simulink model "Inverse7Joint"  (R2023a)
settings: Solver=VariableStepAuto  StartTime=0.0  StopTime=240  RelTol=1e-3
libraries: dspnetwork x2, sldrtlib x1
settings Model: Creator=dr  LastModifiedBy=jeric
settings DebuggingCC: UnconnectedInputMsg=warning  UnconnectedOutputMsg=warning  UnconnectedLineMsg=warning
settings ModelReferenceCC: EnableRefExpFcnMdlSchedulingChecks=on
settings RTWCC: DLArmComputeVersion=19.05

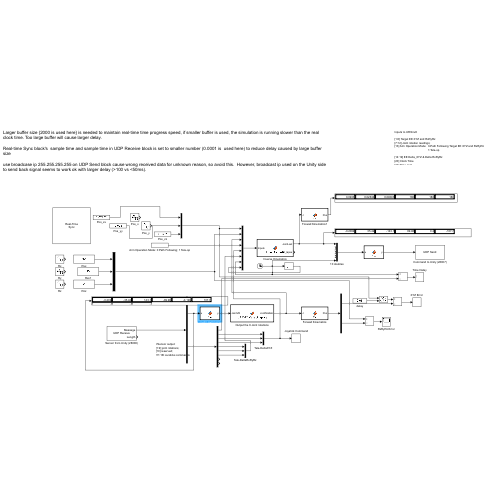
[thumbnail: Simulink's stored preview of the top-level diagram]
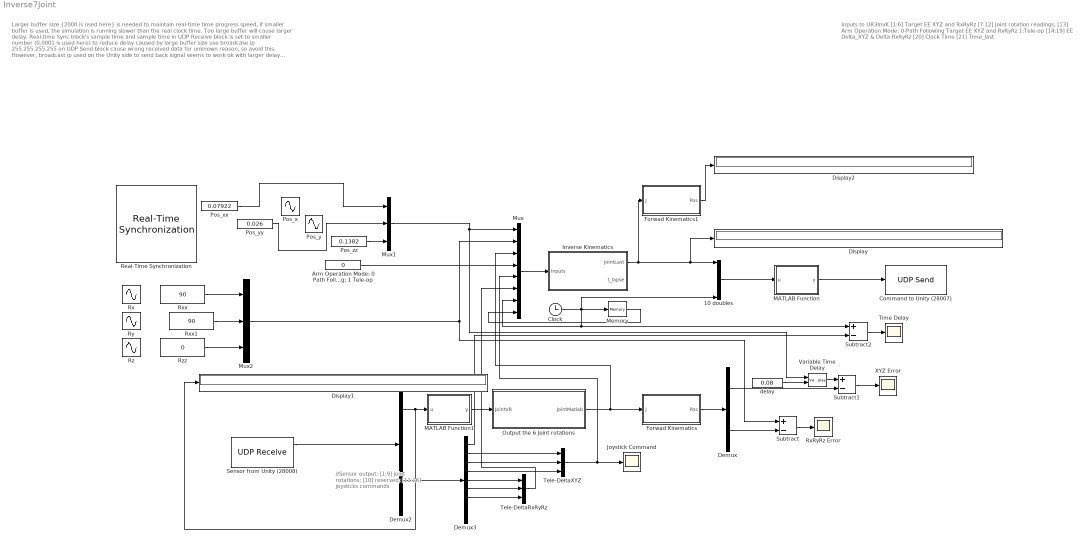
== system Inverse7Joint ==
  note: //Sensor output:
      | [1:9] joint rotations;
      | [10] reserved;
      | [11:16] joysticks commands
  note: Larger buffer size {2000 is used here} is needed to maintain real-time time progress speed, if smaller buffer is used, the simulation is running slower than the real clock time. Too large buffer will cause larger delay.
      |
      | Real-time Sync block's sample time and sample time in UDP Receive block is set to smaller number (0.0001 is used here) to reduce delay caused by large buffer size
      |
      | use broadcase ip 255.255.255.255 on UDP Send block cause wrong received data for unknown reason, so avoid this. However, broadcast ip used on the Unity side to send back signal seems to work ok with larger delay (>100 vs <50ms).
  note: Inputs to UR3InvK
      |
      | [1:6] Target EE XYZ and RxRyRz
      | [7:12] Joint rotation readings;
      | [13] Arm Operation Mode: 	0-Path Following Target EE XYZ and RxRyRz
      | 						1:Tele-op
      |
      | [14:19] EE Delta_XYZ & Delta RxRyRz
      | [20] Clock Time
      | [21] Time_last
  " Joystick Command" : Scope
  10 doubles : Mux  Inputs=5
  Arm Operation Mode: 0 Path Following; 1 Tele-op : Constant  Value=0
  Clock : Clock
  Command to Unity (28007) : dspnetwork/UDP Send  remoteURL='127.0.0.1'  remotePort=28007  localURL='0.0.0.0'  localPortSource=Automatically determine  localPort=-1  sendBufferSize=2500  sampletime=-1  blockPlatform=[]  separateLengthPort=0
  Demux : Demux  Outputs=2
  Demux2 : Demux  Outputs=2
  Demux3 : Demux  Outputs=9
  Display : Display
  Display1 : Display
  Display2 : Display
  Forwad Kinematics : MATLAB Function  TreatAsAtomicUnit=on
  Forwad Kinematics1 : MATLAB Function  TreatAsAtomicUnit=on
  Inverse Kinematics : MATLAB Function  TreatAsAtomicUnit=on
  MATLAB Function : MATLAB Function  TreatAsAtomicUnit=on
  MATLAB Function1 : MATLAB Function  TreatAsAtomicUnit=on
  Memory : Memory  InheritSampleTime=on
  Mux : Mux  Inputs=8
  Mux1 : Mux  Inputs=3
  Mux2 : Mux  Inputs=3
  Output the 6 Joint rotations : MATLAB Function  TreatAsAtomicUnit=on
  Pos_x : Sin  Amplitude=0.15  Bias=.38  Frequency=.0785  Phase=1.57  SampleTime=0.001
  Pos_xx : Constant  Value=0.07922
  Pos_y : Sin  Amplitude=0.2  Frequency=.0785  SampleTime=0.001
  Pos_yy : Constant  Value=0.026
  Pos_zz : Constant  Value=0.1382
  Real-Time Synchronization : sldrtlib/Real-Time Synchronization  SampleTime=0.0001  MaxMissedTicks=10000000  ShowMissedTicks=off  YieldWhenWaiting=on
  Rx : Sin  Amplitude=45  Bias=180  Frequency=.5  SampleTime=0.001
  RxRyRz Error : Scope
  Rxx : Constant  Value=90
  Rxx1 : Constant  Value=90
  Ry : Sin  Amplitude=45  Frequency=.5  SampleTime=0.001
  Rz : Sin  Amplitude=180  Bias=-90  Frequency=1.57  SampleTime=0.001
  Rzz : Constant  Value=0
  Sensor from Unity (28008) : dspnetwork/UDP Receive  localURL='0.0.0.0'  localPort=28008  remoteURL='127.0.0.1'  remotePort=-1  recvBufferSize=2500  dims=18  signalDatatype=double  isComplex=off  isVarSize=off  showBlockingTime=off  blockingTime=0  sampletime=0.0001  blockPlatform=[]
  Subtract : Sum  Inputs=+-
  Subtract1 : Sum  Inputs=+-
  Subtract2 : Sum  Inputs=+-
  Tele-DeltaRxRyRz : Mux  Inputs=3
  Tele-DeltaXYZ : Mux  Inputs=3
  Time Delay : Scope
  Variable Time Delay : VariableTransportDelay  MaximumDelay=10
  XYZ Error : Scope
  delay : Constant  Value=0.08
  wires:
  Mux/1 -> Inverse Kinematics/1(Inputs)
  Subtract/1 -> RxRyRz Error/1
  Output the 6 Joint rotations/1(JointMatlab) -> Mux/3, Forwad Kinematics/1(J)
  Demux/2 -> Subtract/2
  Demux/1 -> Subtract1/2
  Subtract1/1 -> XYZ Error/1
  Mux2/1 -> Mux/2, Subtract/1
  Forwad Kinematics/1(Pos) -> Demux/1
  Clock/1 -> 10 doubles/5, Mux/7, Subtract2/1, Memory/1
  Memory/1 -> Mux/8
  Rxx/1 -> Mux2/1
  Rzz/1 -> Mux2/3
  Mux1/1 -> Variable Time Delay/1, Mux/1
  Sensor from Unity (28008)/1 -> Demux2/1
  Demux2/2 -> Demux3/1
  Demux3/2 -> Tele-DeltaXYZ/1
  Demux3/3 -> Tele-DeltaXYZ/2
  Demux3/4 -> Tele-DeltaXYZ/3
  Demux3/5 -> Tele-DeltaRxRyRz/1
  Demux3/6 -> Tele-DeltaRxRyRz/2
  Demux3/7 -> Tele-DeltaRxRyRz/3
  Tele-DeltaXYZ/1 -> " Joystick Command"/1, Mux/5
  Arm Operation Mode: 0 Path Following; 1 Tele-op/1 -> Mux/4
  Tele-DeltaRxRyRz/1 -> Mux/6
  Subtract2/1 -> Time Delay/1
  Demux3/1 -> Subtract2/2
  Variable Time Delay/1 -> Subtract1/1
  delay/1 -> Variable Time Delay/2
  Rxx1/1 -> Mux2/2
  Pos_zz/1 -> Mux1/3
  Pos_xx/1 -> Mux1/1
  Pos_yy/1 -> Mux1/2
  Forwad Kinematics1/1(Pos) -> Display2/1
  Inverse Kinematics/1(JointLast) -> Forwad Kinematics1/1(J), Display/1, 10 doubles/1
  Demux2/1 -> MATLAB Function1/1(u), Display1/1
  10 doubles/1 -> MATLAB Function/1(u)
  MATLAB Function/1(y) -> Command to Unity (28007)/1
  MATLAB Function1/1(y) -> Output the 6 Joint rotations/1(JointVR)

== matlab function Inverse7Joint/Forwad Kinematics ==
  data: J input; Pos output

function Pos = FK(J)
    Joint = zeros(7,1);
    Pos = zeros(6,1);

    D2R = pi/180;

    for i = 1:6
        Joint(i) = J(i)*D2R;
    end
    Joint(7) = J(7);
    PTool = [0;0;-0.068;1];
    
    dh = [pi 0 0 Joint(1);
          pi/2 0 0 Joint(2);
          0 0.19538 0 Joint(3);
          0 0.16737 -0.0025 Joint(4);
          -pi/2 0 -0.05 Joint(5);
          -pi/2 0 -0.0285 Joint(6)];

 
    T=[1 0 0 0;0 1 0 0; 0 0 1 0; 0 0 0 1];

    for i = 1:6
        T = T*[cos(dh(i,4))              -sin(dh(i,4))             0             dh(i,2);
               sin(dh(i,4))*cos(dh(i,1)) cos(dh(i,4))*cos(dh(i,1)) -sin(dh(i,1)) -sin(dh(i,1))*dh(i,3);
               sin(dh(i,4))*sin(dh(i,1)) cos(dh(i,4))*sin(dh(i,1)) cos(dh(i,1))  cos(dh(i,1))*dh(i,3);
               0                         0                         0             1];
    end
    PTemp = T*PTool;
    Pos(1:3) = PTemp(1:3);

    Pos(4:6) = R2FA(T(1:3,1:3));
    Pos(4:6) = Pos(4:6)/D2R;

function [AX, AY, AZ] = R2FA(R)
    M = 0.0001;
    AY= atan2(-R(3,1), sqrt(R(1,1)^2+R(2,1)^2));
    CAY = cos(AY);

    if abs(CAY)>M
        AZ=atan2(R(2,1)/CAY, R(1,1)/CAY);
        AX=atan2(R(3,2)/CAY, R(3,3)/CAY);
    elseif AY>0
       AY=pi/2;
       AZ=0;
       AX=atan2(R(1,2), R(2,2));
    else
       AY=-pi/2;
       AZ=0; 
       AX=-atan2(R(1,2), R(2,2));
end

== matlab function Inverse7Joint/Forwad Kinematics1 ==
  data: J input; Pos output

function Pos = FK(J)
    Joint = zeros(7,1);
    Pos = zeros(6,1);

    D2R = pi/180;

    for i = 1:6
        Joint(i) = J(i)*D2R;
    end
    Joint(7) = J(7);
    PTool = [0;0;-0.068;1];
    
    dh = [pi 0 0 Joint(1);
          pi/2 0 0 Joint(2);
          0 0.19538 0 Joint(3);
          0 0.16737 -0.0025 Joint(4);
          -pi/2 0 -0.05 Joint(5);
          -pi/2 0 -0.0285 Joint(6)];

 
    T=[1 0 0 0;0 1 0 0; 0 0 1 0; 0 0 0 1];

    for i = 1:6
        T = T*[cos(dh(i,4))              -sin(dh(i,4))             0             dh(i,2);
               sin(dh(i,4))*cos(dh(i,1)) cos(dh(i,4))*cos(dh(i,1)) -sin(dh(i,1)) -sin(dh(i,1))*dh(i,3);
               sin(dh(i,4))*sin(dh(i,1)) cos(dh(i,4))*sin(dh(i,1)) cos(dh(i,1))  cos(dh(i,1))*dh(i,3);
               0                         0                         0             1];
    end
    PTemp = T*PTool;
    Pos(1:3) = PTemp(1:3);

    Pos(4:6) = R2FA(T(1:3,1:3));
    Pos(4:6) = Pos(4:6)/D2R;

function [AX, AY, AZ] = R2FA(R)
    M = 0.0001;
    AY= atan2(-R(3,1), sqrt(R(1,1)^2+R(2,1)^2));
    CAY = cos(AY);

    if abs(CAY)>M
        AZ=atan2(R(2,1)/CAY, R(1,1)/CAY);
        AX=atan2(R(3,2)/CAY, R(3,3)/CAY);
    elseif AY>0
       AY=pi/2;
       AZ=0;
       AX=atan2(R(1,2), R(2,2));
    else
       AY=-pi/2;
       AZ=0; 
       AX=-atan2(R(1,2), R(2,2));
end

== matlab function Inverse7Joint/Inverse Kinematics ==
  data: Inputs input; JointLast output; t_lapse output
function [JointLast, t_lapse]  = LunarArmInvK (Inputs)
persistent  PositionLast  RotationLast;

if isempty(PositionLast)
    PositionLast =zeros(3,1);
end

if isempty(RotationLast)
    RotationLast =zeros(3,1);
end

 
t_lapse = Inputs(20)- Inputs(21);

if Inputs(20) > 0.0 % delay start to make sure sensor data from the VR robot has arrived, during delay, send out the initial joint position 
 
% LEFT  ARM
% This function will generate the joint angle set for each joint on left
% arm based on drawing a circle on XZ plane, radius is RD.
% there are many import parameters is based on physical arm dimensions.
% please contact Dr Robot Inc for further information.

% The demo code is just for 'demo' use.

%cal Jacobian using 5.1.27, page 115, Robot Dyn and Control by Spong
%JInit

steps=5; 

Joint = zeros(6,steps+1);
JointWS = zeros(6,2);
Origin = zeros(3,6);
Axis = zeros(3,6);
PEnd = zeros (3,steps);
Jaco = zeros (6,6);
PTarget = zeros(3, steps+1);
FATarget = zeros(3, steps+1);
ODelta = zeros(3,steps);
WJointLtd = zeros (6,6);
JointLast = zeros (6,1);
RTeleDelta = eye(3,3);
finalPos = zeros(3,1);
finalRxRyRz = zeros(3,1);
PTeleDelta = zeros (3,1);  
Degree2Radian = pi/180;
RxRyRzTeleDelta = zeros(3,1);
RJ5 = zeros(3,3);

%initial joint position
Joint(1,1)= Inputs(7)*Degree2Radian;
Joint(2,1)= Inputs(8)*Degree2Radian;
Joint(3,1)= Inputs(9)*Degree2Radian;
Joint(4,1)= Inputs(10)*Degree2Radian;
Joint(5,1)= Inputs(11)*Degree2Radian;
Joint(6,1)= Inputs(12)*Degree2Radian;

%########################physical dimensions #############################
%Joint limit in degrees
JointLtd=[  -180,   180;
             -205,   25;
            -160,   160;
            -180,   180;
            -180,   180;
            -180,   180];
JointLtdExRate = 50; %Joint ltd avoidance exp increase rate, if this rate is too small, e.g. 10 or 1, it may exceed the limit a bit; 
JointSB=20; % safe zone before reaching joint limit, joint limit avoidance scheme starts action when entering the safe zone. effect grows exponentially
%Convert the safe operation zone (with a boundary of JointSB before the
%limit) from degree into the RAD
for i=1:6
           JointWS(i,1)=(JointLtd(i,1)+JointSB)*Degree2Radian;
           JointWS(i,2)=(JointLtd(i,2)-JointSB)*Degree2Radian;
end
       
T=[1 0 0 0;0 1 0 0; 0 0 1 0; 0 0 0 1]; %INITIAL  Transformation matrix
PTool=[0;0;-0.068;1]; %The Tool or tip position expressed wrt the last frame physical dimension
%Catisian space task weighting, i.e. position and orientation tracking task
%weight, smaller , less significant to track, i.e. by setting WEnd(4,4)
%smaller (e.g. 0.01 while others are 1), the rotation along RX axis will not be tracked precisely.
%!!!!!!!!!!!!!!!!!!!!CHANGE HERE

WEnd=[1 0 0 0 0 0;
    0 1 0 0 0 0;
    0 0 1 0 0 0;
    0 0 0 1 0 0;
    0 0 0 0 1 0;
    0 0 0 0 0 1];           %0.01

%Joint space weighting matrix, larger number will reduce the joint motion,
%i.e. the unit WJoint(6,6)=100, while others are "1" then the joint 6 will
%move very little.
%!!!!!!!!!!!!!!!!!!!!CHANGE HERE
% WJoint=[0.1 0 0 0 0 0;
%         0 0.1 0 0 0 0;
%         0 0 0.1 0 0 0;
%         0 0 0 1 0 0;
%         0 0 0 0 1 0;
%         0 0 0 0 0 1];
WJoint=[1 0 0 0 0 0;
        0 1 0 0 0 0;
        0 0 1 0 0 0;
        0 0 0 1 0 0;
        0 0 0 0 1 0;
        0 0 0 0 0 1];

 
DF2= 0.001; %0.15; %.015; %Damping factor square, larger, slower tracking, bigger tracking error, but more robust to singularity 


for k = 1:steps

    dh = [   pi              0           0           Joint(1,k); 
             pi/2           0           0           Joint(2,k);
             0              0.19538       0           Joint(3,k);
             0              0.16737       -0.0025           Joint(4,k);
             -pi/2            0           -0.05     Joint(5,k);
             -pi/2           0           -0.0285     Joint(6,k)];
 
T=[1 0 0 0;0 1 0 0; 0 0 1 0; 0 0 0 1]; %INITIAL  Transformation matrix

for m=1:6
T=T*[cos(dh(m,4))                    -sin(dh(m,4))                0               dh(m,2)
    sin(dh(m,4))*cos(dh(m,1))   cos(dh(m,4))*cos(dh(m,1))   -sin(dh(m,1))       -sin(dh(m,1))*dh(m,3)
    sin(dh(m,4))*sin(dh(m,1))   cos(dh(m,4))*sin(dh(m,1))   cos(dh(m,1))       cos(dh(m,1))*dh(m,3)
    0                               0                           0               1];
Axis(1:3,m)=T(1:3,3);
Origin(1:3,m)= T(1:3,4);
%if m==5 % copy the second last joint, (before the hand) Rotation
%    RJ5 = T(1:3,1:3);
%end

end

PEndTemp=T*PTool;
PEnd(1:3,k)=PEndTemp(1:3); %tip position in origin frame

%Jacobian upper part , i.e. the linear velocity part
Jaco(1:3,1)= cross (Axis (1:3,1), (PEnd (1:3,k) - Origin(1:3,1)));
Jaco(1:3,2)= cross (Axis (1:3,2), (PEnd (1:3,k)- Origin(1:3,2)));
Jaco(1:3,3)= cross (Axis (1:3,3), (PEnd (1:3,k)- Origin(1:3,3)));
Jaco(1:3,4)= cross (Axis (1:3,4), (PEnd (1:3,k)- Origin(1:3,4)));
Jaco(1:3,5)= cross (Axis (1:3,5), (PEnd (1:3,k)- Origin(1:3,5)));
Jaco(1:3,6)= cross (Axis (1:3,6), (PEnd (1:3,k)- Origin(1:3,6)));

%Jacobian lower part , i.e. the angular velocity part
Jaco(4:6,1)= Axis (1:3,1);
Jaco(4:6,2)= Axis (1:3,2);
Jaco(4:6,3)= Axis (1:3,3);
Jaco(4:6,4)= Axis (1:3,4);
Jaco(4:6,5)= Axis (1:3,5);
Jaco(4:6,6)= Axis (1:3,6);

if k==1 %cal the initial posotition and orientation from the initial joint reading
%target position, should use the sensor reading to calculate the X,Y,Z and
%plan the end effector motion accordingly to avoid rapid movement at start

PInitial    = PEnd(1:3,1);
RInitial    = T(1:3,1:3);
    
%Initialize the tip motion Target 
PTarget(1, 1) = PInitial(1);
PTarget(2, 1) = PInitial(2);
PTarget(3, 1) = PInitial(3) ;

InitialRxRyRZ=R2FixAngle(RInitial);
 
FATarget(1:3,1) = InitialRxRyRZ; %using Fixed-Angle representation page 47, intro to robotics

% set the final target position and RxRyRz
    if Inputs(13) >=1 % 1: tele-operation on end-effector, using Mode switching Initial pos + delat pos as the final target 
        magPosCommand = norm(Inputs(14:16));
        magRotCommand = norm(Inputs(17:19)); 

     if magPosCommand < 0.2  %no motion needed
         PTeleDelta = zeros(3,1);
     else
         PTeleDelta =RInitial*Inputs(14:16)*t_lapse*0.1;
     end

     if magRotCommand < 0.2 %no rotation needed
        RTeleDelta = eye(3,3);
     else
        RxRyRzTeleDelta = Inputs(17:19)*t_lapse*0.5;
        RTeleDelta = FixAngle2R (RxRyRzTeleDelta(1:3));   
     end
        
        finalPos = PositionLast + PTeleDelta;
        finalRxRyRz=R2FixAngle(FixAngle2R(RotationLast*Degree2Radian)*RTeleDelta)*180/pi;
        %finalRxRyRz = Inputs (4:6);
     
    else % =0 path following
        finalPos = Inputs (1:3);
        finalRxRyRz = Inputs (4:6);
    end
end    


%linear planning 
PTarget(1, k+1) = PTarget(1,1) + (finalPos(1)-PTarget(1,1))/steps*k;
PTarget(2, k+1) = PTarget(2,1) + (finalPos(2)-PTarget(2,1))/steps*k ;
PTarget(3, k+1) = PTarget(3,1) + (finalPos(3)-PTarget(3,1))/steps*k;
%PTarget(3, k+1) = PTarget(3,1) - RD - RD*cos(pi+ 2*pi*k/steps);


%planning the orientation motion

FATarget(1,k+1)= finalRxRyRz(1)*Degree2Radian ; 
FATarget(2,k+1)= finalRxRyRz(2)*Degree2Radian ;
FATarget(3,k+1)= finalRxRyRz(3)*Degree2Radian ;

RTarget = FixAngle2R(FATarget(1:3,k+1));

%tip motion delta
PDelta= PTarget(1:3,k+1)-PEnd(1:3,k);
%Rotation error
Rerror = RTarget*(T(1:3,1:3)');
ODelta(1:3,k) = 0.5*[Rerror(3,2)-Rerror(2,3); Rerror(1,3)-Rerror(3,1);Rerror(2,1)-Rerror(1,2)];

%Least square pseudo inverse of J
JacoP=Jaco(1:6,1:6);
%Jw=transpose(JacoP)*inv(JacoP*transpose(JacoP)+ DF2*eye(6));


%Joint limit avoidance
for i=1:6
    if Joint(i,k)>JointWS(i,2)
        JointOver= Joint(i,k)-JointWS(i,2);
    elseif     Joint(i,k) <JointWS(i,1)
        JointOver= JointWS(i,1)-Joint(i,k) ;
    else
       JointOver=0;     
   end   
WJointLtd(i,i)=WJoint(i,i)*exp(JointLtdExRate*JointOver); %Augment the WJoint weighting matrix with the Joint Limit Avoidance, closer to the limit, the Weighting unit will increase exponentially, and leading to smaller velocity till stop, therefore avoiding exceeding the limit
end

Jw=inv(transpose(JacoP)*WEnd*JacoP+ DF2*(WJointLtd))*transpose(JacoP)*WEnd;

%conJ=cond(JacoP)
%Jw=inv(Jaco);
%inverse kinematic of delta joint motion 

JDelta= Jw*[PDelta;ODelta(1:3,k)]; 

%orientation only
%Jw=W1*transpose(Jaco(4:6,1:6))*inv(Jaco(4:6,1:6)*W1*transpose(Jaco(4:6,1:6)));
%JDelta= Jw*[ODelta];

%with error on joint trackin
%Joint(1:6,k+2)=Joint(1:6,k+1)+JDelta + dot (JDelta, [0.5*(rand-0.5);0.5*(rand-0.5);0.5*(rand-0.5);0.5*(rand-0.5);0.2*(rand-0.5);0.2*(rand-0.5)]);
%here is what the robot arm controller should do: drive the arm to the
%position we need:
Joint(1:6,k+1)=Joint(1:6,k)+JDelta; 
end


JointLast(1:6) = Joint(1:6,k+1)/Degree2Radian;
PositionLast =  finalPos; %storrage of last pos target command 
RotationLast = finalRxRyRz;

else
    %initial position
    %JointLast = [0, 45,90, -45, 90, 0]';
    JointLast = [0, -135,135,90,0,0]';
    PositionLast =[0.07922, 0.094, 0.1382]';
    RotationLast = [90,90,0]';
end
 

function AxAyAZ= R2FixAngle(R) 

MINA=0.0001; %minimun we consider to be 0 degree

AY= atan2(-R(3,1), sqrt(R(1,1)^2+R(2,1)^2));

CAY=cos(AY);

if abs(CAY)>MINA
    AZ=atan2(R(2,1)/CAY, R(1,1)/CAY);
    AX=atan2(R(3,2)/CAY, R(3,3)/CAY);
elseif AY>0 % AY=90 degree
   AY=pi/2;
   AZ=0; %this is a convention to choose AZ to be zero, see page 47
   AX=atan2(R(1,2), R(2,2));
else  % AY=-90 degree
   AY=-pi/2;
   AZ=0; %this is a convention to choose AZ to be zero, see page 47
   AX=-atan2(R(1,2), R(2,2));
end
AxAyAZ = [AX AY AZ]';

%Fixed Angle representation page 45, intro to robotics
%Definition: Describing the orientation of frame B is as follows:
%start  with the frame coincident with a known reference frame A. First
%rotate B about axis XA by an angle AngleX, then rotate about YA by an
%angle AngleY, and then rotate about ZA by an angle AngleZ.

function [R]= FixAngle2R(AngleXYZ) 

cX  = cos (AngleXYZ(1));
sX  =   sin(AngleXYZ(1));
cY  =   cos (AngleXYZ(2));
sY  =   sin(AngleXYZ(2));
cZ  =   cos (AngleXYZ(3));
sZ  =   sin(AngleXYZ(3));

R=[cZ*cY cZ*sY*sX-sZ*cX cZ*sY*cX+sZ*sX;
   sZ*cY sZ*sY*sX+cZ*cX sZ*sY*cX-cZ*sX;
   -s

== matlab function Inverse7Joint/MATLAB Function ==
  data: u input; y output
function y = fcn(u)

y = [u(1); -u(2 : 6); u(7 : 10)];

== matlab function Inverse7Joint/MATLAB Function1 ==
  data: u input; y output
function y = fcn(u)

y = [u(1); -u(2 : 6)];

== matlab function Inverse7Joint/Output the 6 Joint rotations ==
  data: JointVR input; JointMatlab output
function JointMatlab  = UR3VR2MatlabMaping(JointVR)
JointMatlab  = zeros (6,1);
JointMatlab(1:6) = JointVR(1:6);
